simulink model "controller_incremental"  (R2023b)
settings: Solver=VariableStepAuto  StartTime=0.0  StopTime=10  FixedStep=0.005  RelTol=1e-3  EnableMultiTasking=on
values from neighbouring files (symbols this model uses):
  Ts = 0.005    [lqi_controller_incremental.m]
undefined symbols (not defined in the file or in its folder): DiscIntNeverNeededParam, K
libraries: simulink_extras x2
settings Model: ExtModeTrigDuration=10  Creator=paoli  LastModifiedBy=paoli
settings OptimizationCC: DefaultParameterBehavior=Inlined  EnhancedBackFolding=on  PassReuseOutputArgsAs=Individual arguments  ZeroExternalMemoryAtStartup=off  ZeroInternalMemoryAtStartup=off  MaxStackSize=64  OptimizeBlockOrder=speed  DifferentSizesBufferReuse=on  OptimizationCustomize=off  EfficientTunableParamExpr=on
settings DebuggingCC: ParameterTunabilityLossMsg=error
settings HardwareCC: ProdBitPerPointer=32  ProdBitPerSizeT=32  ProdBitPerPtrDiffT=32  ProdLargestAtomicInteger=Long  ProdLargestAtomicFloat=Double  ProdWordSize=32  ProdLongLongMode=on  ProdHWDeviceType=ARM Compatible->ARM Cortex
settings SFSimCC: MATLABDynamicMemAlloc=off
settings RTWCC: Description=Embedded Coder  SystemTargetFile=ert.tlc  TemplateMakefile=ert_default_tmf  Toolchain=GNU Tools for ARM Embedded Processors
settings CodeAppCC: ForceParamTrailComments=on  IgnoreCustomStorageClasses=off  OperatorAnnotations=on  SimulinkDataObjDesc=on  SFDataObjDesc=on  InsertBlockDesc=on
settings ERTTargetCC: SupportContinuousTime=on  ExtModeTransport=3  ExtModeStaticAlloc=on  ExtModeStaticAllocSize=2000  ExtModeMexFile=ext_xcp  ExtModeIntrfLevel=Level2 - Open  InlinedParameterPlacement=NonHierarchical  ERTCustomFileTemplate=example_file_process.tlc

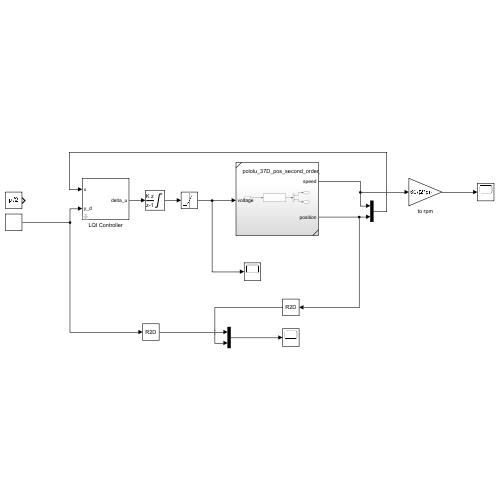
[thumbnail: Simulink's stored preview of the top-level diagram]
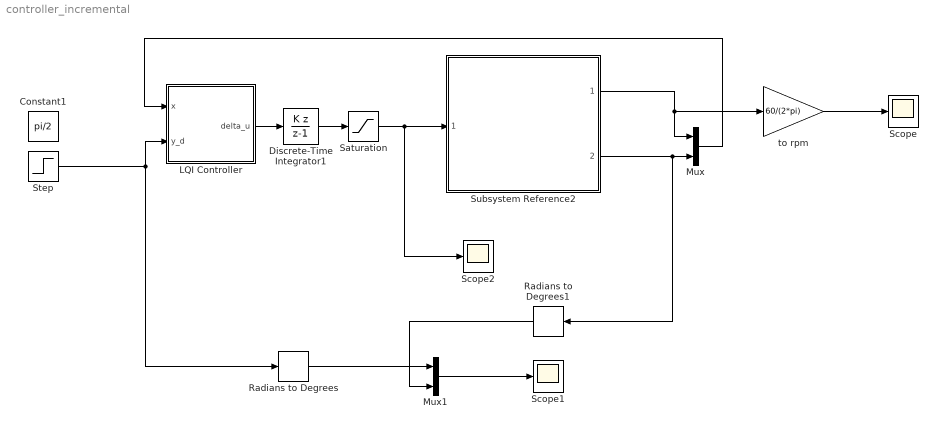
== system controller_incremental ==
  Constant1 : Constant  Value=pi/2
  Discrete-Time Integrator1 : DiscreteIntegrator  IntegratorMethod=Accumulation: Backward Euler  SampleTime=Ts  LimitOutput=on  UpperSaturationLimit=12  LowerSaturationLimit=-12  ICPrevOutput=DiscIntNeverNeededParam  ICPrevScaledInput=DiscIntNeverNeededParam
  LQI Controller : Subsystem  mask{Ts=0.005}
  Mux : Mux  Inputs=2
  Mux1 : Mux  Inputs=2
  Radians to Degrees : simulink_extras/Transformations/Radians to Degrees
  Radians to Degrees1 : simulink_extras/Transformations/Radians to Degrees
  Saturation : Saturate  UpperLimit=12  LowerLimit=-12
  Scope : Scope
  Scope1 : Scope
  Scope2 : Scope
  Step : Step  Time=5  Before=pi  After=2*pi  SampleTime=0
  Subsystem Reference2 : Subsystem  ReferencedSubsystem=pololu_37D_pos_second_order_discrete
  to rpm : Gain  Gain=60/(2*pi)
  wires:
  Mux/1 -> LQI Controller/1(x)
  Subsystem Reference2/1 -> Mux/1, to rpm/1
  Subsystem Reference2/2 -> Radians to Degrees1/1, Mux/2
  to rpm/1 -> Scope/1
  Step/1 -> Radians to Degrees/1, LQI Controller/2(y_d)
  Mux1/1 -> Scope1/1
  Radians to Degrees/1 -> Mux1/1
  Radians to Degrees1/1 -> Mux1/2
  Saturation/1 -> Subsystem Reference2/1, Scope2/1
  LQI Controller/1(delta_u) -> Discrete-Time Integrator1/1
  Discrete-Time Integrator1/1 -> Saturation/1

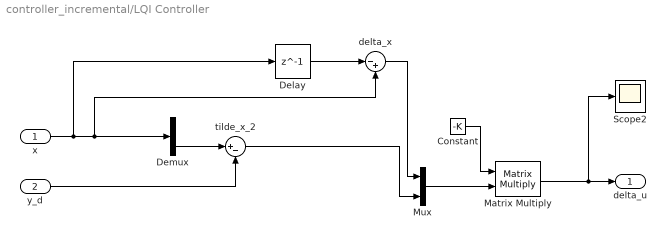
== system controller_incremental/LQI Controller ==
  x : Inport  SampleTime=Ts
  y_d : Inport  Port=2  SampleTime=Ts
  Constant : Constant  Value=-K  VectorParams1D=off
  Delay : Delay  DelayLength=1  InitialCondition=[0;0]  SampleTime=Ts
  Demux : Demux  Outputs=2
  Matrix Multiply : Product  Multiplication=Matrix(*)
  Mux : Mux  Inputs=2
  Scope2 : Scope
  delta_x : Sum  Inputs=|-+
  tilde_x_2 : Sum  Inputs=|+-
  delta_u : Outport  SampleTime=Ts
  wires:
  x/1 -> Delay/1, delta_x/2, Demux/1
  Mux/1 -> Matrix Multiply/2
  Demux/2 -> tilde_x_2/1
  y_d/1 -> tilde_x_2/2
  Delay/1 -> delta_x/1
  tilde_x_2/1 -> Mux/2
  Matrix Multiply/1 -> Scope2/1, delta_u/1
  Constant/1 -> Matrix Multiply/1
  delta_x/1 -> Mux/1
